simulink subsystem "Led"  (R2023b)
settings: Solver=VariableStepAuto  StartTime=0.0  StopTime=10.0  RelTol=1e-3
libraries: arduinolib x3, simulink x1
settings Model: Creator=Usuario_UMA  LastModifiedBy=Usuario

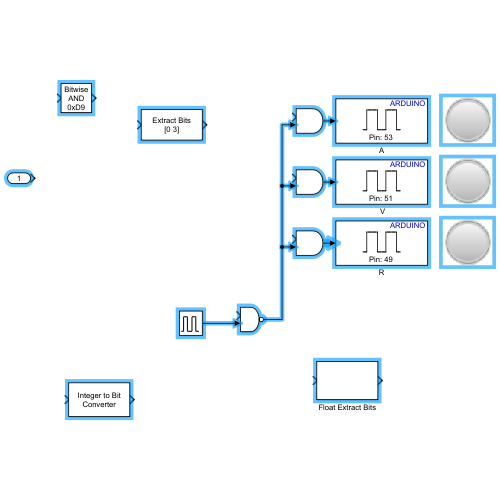
[thumbnail: Simulink's stored preview of the top-level diagram]
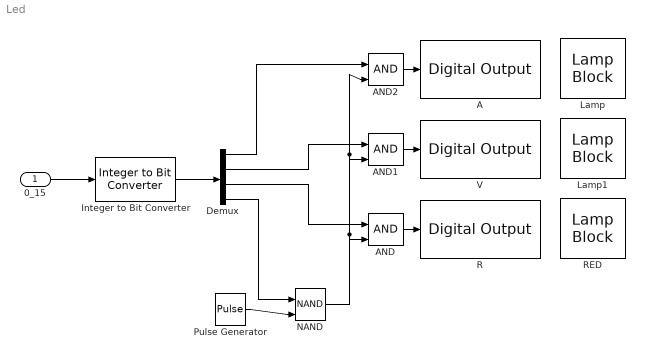
== system Led ==
  0_15 : Inport
  " V" : arduinolib/Digital Output  pinNumber=51  Direction=output  blockPlatform=arduino
  A : arduinolib/Digital Output  pinNumber=53  Direction=output  blockPlatform=arduino
  AND : Logic  IconShape=distinctive  AllPortsSameDT=off  OutDataTypeStr=boolean
  AND1 : Logic  IconShape=distinctive  AllPortsSameDT=off  OutDataTypeStr=boolean
  AND2 : Logic  IconShape=distinctive  AllPortsSameDT=off  OutDataTypeStr=boolean
  Demux : Demux
  Integer to Bit Converter : simulink/Logic and Bit Operations/Integer to Bit Converter  nbits=4  signedInputValues=Unsigned  bitOrder=LSB first  outDtype=boolean
      settings: LibrarySourceBlock=|
      | commutil2/Integer to Bit
      | Converter
  Lamp : LampBlock  LabelPosition=Hide
  Lamp1 : LampBlock  LabelPosition=Hide
  NAND : Logic  Operator=NAND  IconShape=distinctive  AllPortsSameDT=off  OutDataTypeStr=boolean
  Pulse Generator : DiscretePulseGenerator  PulseType=Time based  Period=1  PulseWidth=50
  R : arduinolib/Digital Output  pinNumber=49  Direction=output  blockPlatform=arduino
  RED : LampBlock  LabelPosition=Hide
  wires:
  Pulse Generator/1 -> NAND/2
  NAND/1 -> AND2/2, AND1/2, AND/2
  AND1/1 -> " V"/1
  AND2/1 -> A/1
  AND/1 -> R/1
  0_15/1 -> Integer to Bit Converter/1
  Integer to Bit Converter/1 -> Demux/1
  Demux/2 -> AND1/1
  Demux/3 -> AND/1
  Demux/1 -> AND2/1
  Demux/4 -> NAND/1
